simulink model "interp_2"  (Simulink 4.00)
settings: Solver=ode45  StartTime=0.0  StopTime=10.0  RelTol=1e-3
libraries: simulink3 x5
settings Model: LastModifiedBy=Administrator  BlockReductionOpt=off

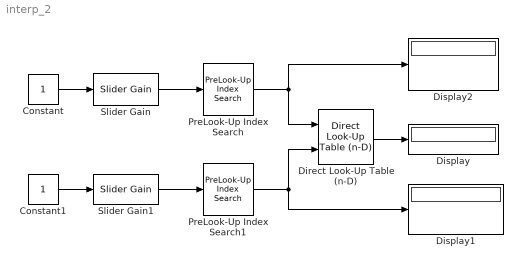
== system interp_2 ==
  Constant : Constant  Value=1
  Constant1 : Constant  Value=1
  Direct Look-Up Table (n-D) : simulink3/Functions & Tables/Direct Look-Up Table (n-D)  maskTabDims=2  explicitNumDims=1  outDims=Element  tabIsInput=off  mxTable=[sqrt([1:10]'*[1:10])]  clipFlag=Warning
  Display : Display
      settings: Format=short
  Display1 : Display
      settings: Format=short
  Display2 : Display
      settings: Format=short
  PreLook-Up Index Search : simulink3/Functions & Tables/PreLook-Up Index Search  bpData=[5:14]  searchMode=Binary Search  cacheBpFlag=off  outputFlag=off  extrapMode=Linear Extrapolation  rangeErrorMode=None
  PreLook-Up Index Search1 : simulink3/Functions & Tables/PreLook-Up Index Search  bpData=[20:10:110]  searchMode=Binary Search  cacheBpFlag=off  outputFlag=off  extrapMode=Linear Extrapolation  rangeErrorMode=None
  Slider Gain : simulink3/Math/Slider Gain  low=5  gain=8.48  high=14
  Slider Gain1 : simulink3/Math/Slider Gain  low=20  gain=76.34  high=110
  wires:
  PreLook-Up Index Search/1 -> Direct Look-Up Table (n-D)/1, Display2/1
  PreLook-Up Index Search1/1 -> Direct Look-Up Table (n-D)/2, Display1/1
  Direct Look-Up Table (n-D)/1 -> Display/1
  Constant/1 -> Slider Gain/1
  Slider Gain/1 -> PreLook-Up Index Search/1
  Constant1/1 -> Slider Gain1/1
  Slider Gain1/1 -> PreLook-Up Index Search1/1
